simulink model "p2b1"  (R2023b)
settings: Solver=VariableStepAuto  StartTime=0.0  StopTime=10.0  RelTol=1e-3
settings Model: Creator=tanvi  LastModifiedBy=tanvi

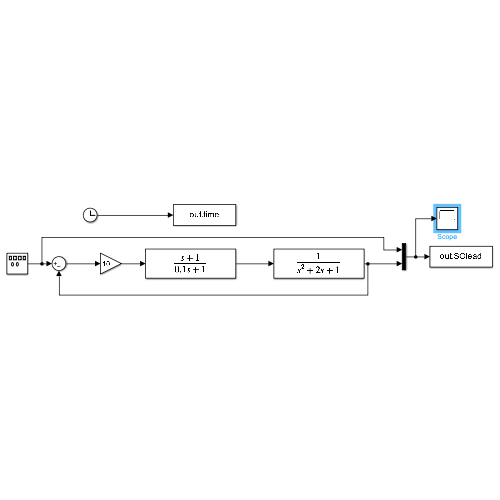
[thumbnail: Simulink's stored preview of the top-level diagram]
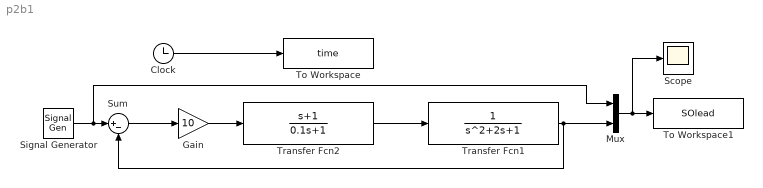
== system p2b1 ==
  Clock : Clock
  Gain : Gain  Gain=10
  Mux : Mux  Inputs=2
  Scope : Scope
  Signal Generator : SignalGenerator  WaveForm=square  Frequency=0.15
  Sum : Sum  Inputs=|+-
  To Workspace : ToWorkspace  VariableName=time  SampleTime=-1
  To Workspace1 : ToWorkspace  VariableName=SOlead  SampleTime=-1
  Transfer Fcn1 : TransferFcn
  Transfer Fcn2 : TransferFcn  Numerator=[1 1]  Denominator=[0.1 1]
  wires:
  Clock/1 -> To Workspace/1
  Mux/1 -> To Workspace1/1, Scope/1
  Signal Generator/1 -> Mux/1, Sum/1
  Sum/1 -> Gain/1
  Gain/1 -> Transfer Fcn2/1
  Transfer Fcn2/1 -> Transfer Fcn1/1
  Transfer Fcn1/1 -> Sum/2, Mux/2
